simulink model "flightcode"  (R2016b)
settings: Solver=VariableStepAuto  StartTime=0.0  StopTime=10.0  FixedStep=MPCSampleTime  RelTol=1e-3  EnableMultiTasking=on
settings Model: SimulationMode=accelerator  Creator=austinmurch  LastModifiedBy=UAVLAB
settings DataIOCC: LimitDataPoints=on  SaveFormat=Array  SignalLoggingSaveFormat=ModelDataLogs
settings OptimizationCC: DefaultParameterBehavior=Inlined  ExpressionDepthLimit=2147483647  LifeSpan=inf  SimCompilerOptimization=on
settings DebuggingCC: SolverPrmCheckMsg=warning  FcnCallInpInsideContextMsg=warning  StateNameClashWarn=warning  SFUnexpectedBacktrackingDiag=warning  SFNoUnconditionalDefaultTransitionDiag=warning  SFExecutionAtInitializationDiag=none
settings HardwareCC: ProdBitPerPointer=32  ProdBitPerSizeT=32  ProdBitPerPtrDiffT=32  ProdLargestAtomicInteger=Long  ProdLargestAtomicFloat=Double  ProdEndianess=BigEndian  ProdWordSize=32  ProdHWDeviceType=Freescale->32-bit PowerPC
settings ModelReferenceCC: ModelReferenceNumInstancesAllowed=Single  PropagateSignalLabelsOutOfModel=off
settings GRTTargetCC: TargetLangStandard=C89/C90 (ANSI)  GeneratePreprocessorConditionals=Disable all  CombineOutputUpdateFcns=off  GRTInterface=on
settings ConfigComp: CovMetricSettings=dw  CovHtmlReporting=on  CovSaveCumulativeToWorkspaceVar=on  CovSaveSingleToWorkspaceVar=on  CovExternalEMLEnable=off

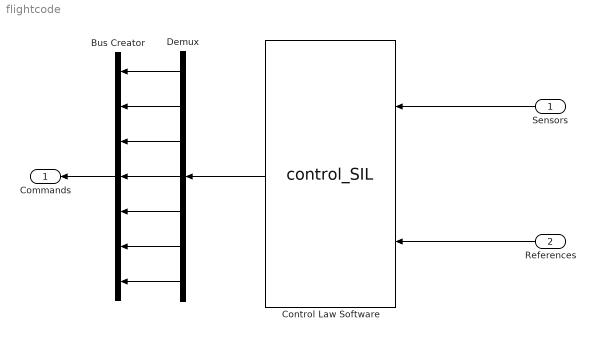
== system flightcode ==
  Sensors : Inport  OutDataTypeStr=Bus: Sensors
  References : Inport  Port=2  OutDataTypeStr=Bus: Refs
  Bus Creator : BusCreator  Inputs=7  OutDataTypeStr=Bus: Commands
      settings: InheritFromInputs=off
  Control Law Software : S-Function  FunctionName=control_SIL  Parameters=SampleTime  SFunctionDeploymentMode=off  EnableBusSupport=off
  Demux : Demux  Outputs=7
  Commands : Outport  OutDataTypeStr=Bus: Commands
  wires:
  Sensors/1 -> Control Law Software/1
  References/1 -> Control Law Software/2
  Bus Creator/1 -> Commands/1
  Demux/7 -> Bus Creator/7
  Demux/6 -> Bus Creator/6
  Demux/5 -> Bus Creator/5
  Demux/4 -> Bus Creator/4
  Demux/3 -> Bus Creator/3
  Demux/2 -> Bus Creator/2
  Demux/1 -> Bus Creator/1
  Control Law Software/1 -> Demux/1
